simulink library "lib_Convection_MixedIncompFlatPlateBL"  (R2015a)
settings: Solver=ode45  StartTime=0.0  StopTime=10.0  RelTol=1e-3
libraries: lib_Convection_LamIncompFlatPlateBL x1
settings Model: Creator=jlkratz  LastModifiedBy=jlkratz

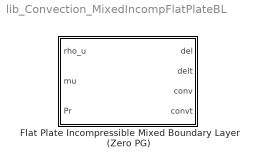
== system lib_Convection_MixedIncompFlatPlateBL ==
  Flat Plate Incompressible Mixed Boundary Layer (Zero PG) : Subsystem  mask(TSAT: Flat Plate Incompressible Mixed Boundary Layer (Zero PG)){x_M=[0.01:0.1:5], BN_M=double(gcb), Retr_M=5000000, xtrip_M=inf}
      mask prompts: x_M "x_M - Local position from the leading edge"; BN_M "BN_M - Block Name"; Retr_M "Retr_M - Transition Reynolds number"; xtrip_M "xtrip_M - Location of a boundary layer trip (inf if none exists)"
      mask help:
      | This block approximates the boundary layer and thermal boundary layer thicknesses of incompressible mixed flow over a flat plate with a pressure gradient of 0. It determines the transition location by the transition Reynolds number or a trip location, whichever is closer to the leading edge. The boundary layer upstream of the transition location is calculated based on the laminar boundary layer solution while downstream the turbulent solution is used. The turbulent solution is shifted such that it intersects the laminar solution at the transition location.
      |
      | For more information see the block help menu.
      mask Help: web(which('Convection_TSAT_MixedIncompFlatPlateBL.html'),'-helpbrowser')
      mask DialogControl Container3 Prompt: Parameters
      mask DialogControl Container5 Prompt: Transition

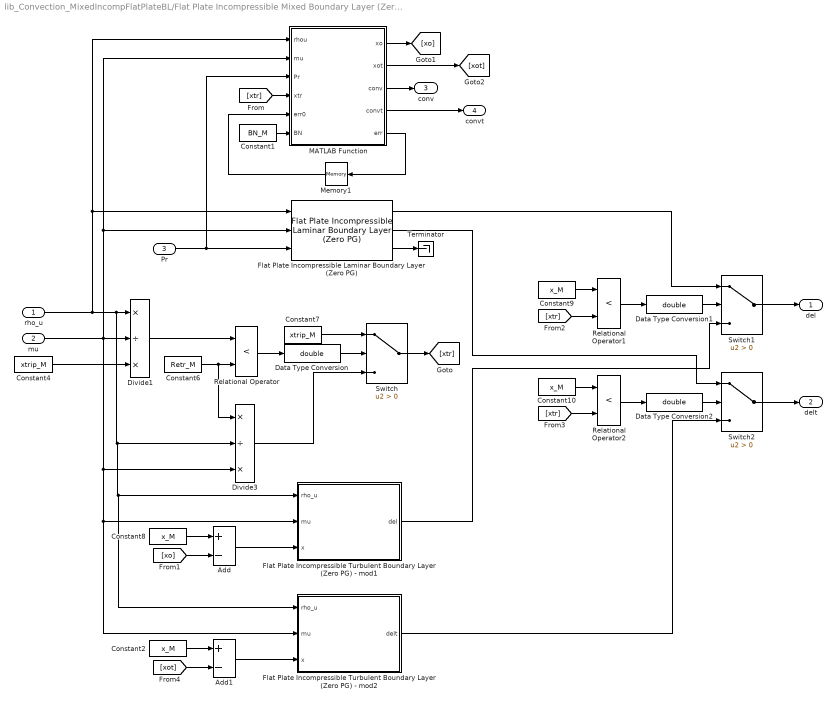
== system lib_Convection_MixedIncompFlatPlateBL/Flat Plate Incompressible Mixed Boundary Layer (Zero PG) ==
  rho_u : Inport
  mu : Inport  Port=2
  Pr : Inport  Port=3
  Add : Sum  Inputs=+-
  Add1 : Sum  Inputs=+-
  Constant1 : Constant  Value=BN_M
  Constant{2,8..10} (4 alike) : Constant  Value=x_M
  Constant4 : Constant  Value=xtrip_M
  Constant6 : Constant  Value=Retr_M
  Constant7 : Constant  Value=xtrip_M
  Data Type Conversion : DataTypeConversion  OutDataTypeStr=double
  Data Type Conversion1 : DataTypeConversion  OutDataTypeStr=double
  Data Type Conversion2 : DataTypeConversion  OutDataTypeStr=double
  Divide1 : Product  Inputs=*/*
  Divide3 : Product  Inputs=*/*
  Flat Plate Incompressible Laminar Boundary Layer (Zero PG) : lib_Convection_LamIncompFlatPlateBL/Flat Plate Incompressible  Laminar Boundary Layer (Zero PG)  Retr_M=Retr_M  x_M=x_M
  Flat Plate Incompressible Turbulent Boundary Layer (Zero PG) - mod1 : Subsystem  mask(TSAT: Flat Plate Incompressible Turbulent Boundary Layer (Zero PG)){x_M=1}
      mask prompts: x_M "x_M - Local position from the leading edge"
      mask help: This block approximates the boundary layer and thermal boundary layer thicknesses of incompressible turbulent flow over a flat plate with a pressure gradient of 0.
      mask Help: web(which('Convection_TSAT_TurbIncompFlatPlateBL.html'),'-helpbrowser')
      mask DialogControl Container3 Prompt: Parameters
  Flat Plate Incompressible Turbulent Boundary Layer (Zero PG) - mod2 : Subsystem  mask(TSAT: Flat Plate Incompressible Turbulent Boundary Layer (Zero PG)){x_M=1}
      mask prompts: x_M "x_M - Local position from the leading edge"
      mask help: This block approximates the boundary layer and thermal boundary layer thicknesses of incompressible turbulent flow over a flat plate with a pressure gradient of 0.
      mask Help: web(which('Convection_TSAT_TurbIncompFlatPlateBL.html'),'-helpbrowser')
      mask DialogControl Container3 Prompt: Parameters
  MATLAB Function : MATLAB Function  TreatAsAtomicUnit=on
  Memory1 : Memory  X0=zeros(1,9)
  Relational Operator : RelationalOperator  Operator=<  OutDataTypeStr=boolean
  Relational Operator1 : RelationalOperator  Operator=<  OutDataTypeStr=boolean
  Relational Operator2 : RelationalOperator  Operator=<  OutDataTypeStr=boolean
  Switch : Switch  Criteria=u2 > Threshold
  Switch1 : Switch  Criteria=u2 > Threshold
  Switch2 : Switch  Criteria=u2 > Threshold
  Terminator : Terminator
  del : Outport
  delt : Outport  Port=2
  conv : Outport  Port=3
  convt : Outport  Port=4
  wires:
  Add1/1 -> Flat Plate Incompressible Turbulent Boundary Layer (Zero PG) - mod2/3(x)
  [xot] -> Add1/2
  Constant2/1 -> Add1/1
  MATLAB Function/4(convt) -> convt/1
  MATLAB Function/2(xot) -> [xot]
  Memory1/1 -> MATLAB Function/5(err0)
  MATLAB Function/3(conv) -> conv/1
  MATLAB Function/1(xo) -> [xo]
  [xtr] -> MATLAB Function/4(xtr)
  Constant1/1 -> MATLAB Function/6(BN)
  MATLAB Function/5(err) -> Memory1/1
  Switch2/1 -> delt/1
  Switch1/1 -> del/1
  Flat Plate Incompressible Turbulent Boundary Layer (Zero PG) - mod2/1(delt) -> Switch2/3
  Flat Plate Incompressible Turbulent Boundary Layer (Zero PG) - mod1/1(del) -> Switch1/3
  Flat Plate Incompressible Laminar Boundary Layer (Zero PG)/2 -> Switch2/1
  [xtr] -> Relational Operator2/2
  Constant10/1 -> Relational Operator2/1
  Relational Operator2/1 -> Data Type Conversion2/1
  Data Type Conversion2/1 -> Switch2/2
  Flat Plate Incompressible Laminar Boundary Layer (Zero PG)/1 -> Switch1/1
  [xtr] -> Relational Operator1/2
  Constant9/1 -> Relational Operator1/1
  Relational Operator1/1 -> Data Type Conversion1/1
  Data Type Conversion1/1 -> Switch1/2
  Add/1 -> Flat Plate Incompressible Turbulent Boundary Layer (Zero PG) - mod1/3(x)
  [xo] -> Add/2
  Constant8/1 -> Add/1
  Flat Plate Incompressible Laminar Boundary Layer (Zero PG)/3 -> Terminator/1
  Pr/1 -> Flat Plate Incompressible Laminar Boundary Layer (Zero PG)/3, MATLAB Function/3(Pr)
  Divide3/1 -> Switch/3
  Switch/1 -> [xtr]
  Constant7/1 -> Switch/1
  Data Type Conversion/1 -> Switch/2
  Relational Operator/1 -> Data Type Conversion/1
  Constant6/1 -> Relational Operator/2, Divide3/1
  Divide1/1 -> Relational Operator/1
  Constant4/1 -> Divide1/3
  mu/1 -> Divide3/3, Flat Plate Incompressible Turbulent Boundary Layer (Zero PG) - mod1/2(mu), Flat Plate Incompressible Turbulent Boundary Layer (Zero PG) - mod2/2(mu), Flat Plate Incompressible Laminar Boundary Layer (Zero PG)/2, MATLAB Function/2(mu), Divide1/2
  rho_u/1 -> Flat Plate Incompressible Laminar Boundary Layer (Zero PG)/1, MATLAB Function/1(rhou), Divide1/1, Divide3/2, Flat Plate Incompressible Turbulent Boundary Layer (Zero PG) - mod1/1(rho_u), Flat Plate Incompressible Turbulent Boundary Layer (Zero PG) - mod2/1(rho_u)

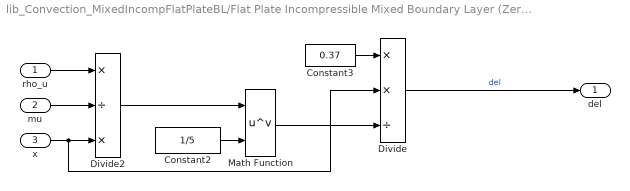
== system lib_Convection_MixedIncompFlatPlateBL/Flat Plate Incompressible Mixed Boundary Layer (Zero PG)/Flat Plate Incompressible Turbulent Boundary Layer (Zero PG) - mod1 ==
  rho_u : Inport
  mu : Inport  Port=2
  x : Inport  Port=3
  Constant2 : Constant  Value=1/5
  Constant3 : Constant  Value=0.37
  Divide : Product  Inputs=**/
  Divide2 : Product  Inputs=*/*
  Math Function : Math  Operator=pow  SaturateOnIntegerOverflow=on
  del : Outport
  wires:
  Divide2/1 -> Math Function/1
  mu/1 -> Divide2/2
  rho_u/1 -> Divide2/1
  x/1 -> Divide2/3, Divide/2
  Constant3/1 -> Divide/1
  Constant2/1 -> Math Function/2
  Math Function/1 -> Divide/3
  Divide/1 -> del/1  "del"

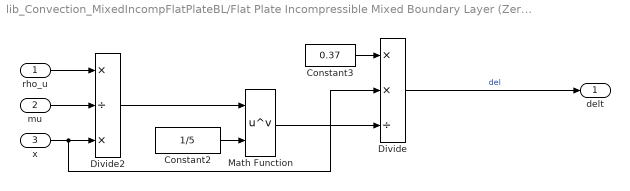
== system lib_Convection_MixedIncompFlatPlateBL/Flat Plate Incompressible Mixed Boundary Layer (Zero PG)/Flat Plate Incompressible Turbulent Boundary Layer (Zero PG) - mod2 ==
  rho_u : Inport
  mu : Inport  Port=2
  x : Inport  Port=3
  Constant2 : Constant  Value=1/5
  Constant3 : Constant  Value=0.37
  Divide : Product  Inputs=**/
  Divide2 : Product  Inputs=*/*
  Math Function : Math  Operator=pow  SaturateOnIntegerOverflow=on
  delt : Outport
  wires:
  Divide/1 -> delt/1  "del"
  Math Function/1 -> Divide/3
  Constant2/1 -> Math Function/2
  Constant3/1 -> Divide/1
  x/1 -> Divide/2, Divide2/3
  rho_u/1 -> Divide2/1
  mu/1 -> Divide2/2
  Divide2/1 -> Math Function/1

== matlab function lib_Convection_MixedIncompFlatPlateBL/Flat Plate Incompressible Mixed Boundary Layer (Zero PG)/MATLAB Function ==
  data: rhou input; xo output; xot output; mu input; Pr input; xtr input; err0 input; BN input; conv output; convt output; err output
function [xo,xot,conv,convt,err] = TransitionXo(rhou,mu,Pr,xtr,err0,BN)
%#codegen

%Warning/Error Check
err = err0;
errNum = 1;
%rhou is a scalar?
if max(size(rhou)) ~= 1 && err0(errNum) ~= 1
    fprintf('warning in %s: rho_u must be a scalar\n',char(BN));
    err(errNum) = 1;
end
errNum = errNum + 1;
%mu is a scalar?
if min(size(mu)) ~= 1 && err0(errNum) ~= 1
    fprintf('warning in %s: mu must be a scalar\n',char(BN));
    err(errNum) = 1;
end
errNum = errNum + 1;
%xtr is a scalar?
if min(size(xtr)) ~= 1 && err0(errNum) ~= 1
    fprintf('warning in %s: xtr must be a scalar\n',char(BN));
    err(errNum) = 1;
end
errNum = errNum + 1;
%rhou is real positive?
if (isreal(rhou) ~= 1 || rhou < 0) && err0(errNum) ~= 1
    fprintf('warning in %s: rho_u must be a real positive number\n',char(BN));
    err(errNum) = 1;
end
errNum = errNum + 1;
%mu is real positive?
if (isreal(mu) ~= 1 || mu < 0) && err0(errNum) ~= 1
    fprintf('warning in %s: mu must be a real positive number\n',char(BN));
    err(errNum) = 1;
end
errNum = errNum + 1;
%xtr is real positive?
if (isreal(xtr) ~= 1 || xtr < 0) && err0(errNum) ~= 1
    fprintf('warning in %s: xtr must be a real positive number\n',char(BN));
    err(errNum) = 1;
end
errNum = errNum + 1;
%rhou has all finite elements?
if (isnan(rhou) > 0 || isinf(rhou) > 0) && err0(errNum) ~= 1
    fprintf('warning in %s: rho_u must have finite value\n',char(BN));
    err(errNum) = 1;
end
errNum = errNum + 1;
%eoD has all finite elements?
if (isnan(mu) > 0 || isinf(mu) > 0) && err0(errNum) ~= 1
    fprintf('warning in %s: mu must have finite value\n',char(BN));
    err(errNum) = 1;
end
%eoD has all finite elements?
if (isnan(xtr) > 0 || isinf(xtr) > 0) && err0(errNum) ~= 1
    fprintf('warning in %s: xtr must have finite value\n',char(BN));
    err(errNum) = 1;
end

%Solve the Colebrook Correlation using the Secant Root Method
Err = 0.000001;
imax = 1000;

%Boundary Layer
Xa = 0.79*xtr;
Xb = 0.83*xtr;
conv = 0;
Xs = 0;
for i = 1:imax %Number iterations is specified by user
    FunXb = 5*xtr*(rhou*xtr/mu)^(-1/2) - 0.37*(xtr-Xb)*(rhou*(xtr-Xb)/mu)^(-1/5); %Value function at Xb is calculated
    FunXa = 5*xtr*(rhou*xtr/mu)^(-1/2) - 0.37*(xtr-Xa)*(rhou*(xtr-Xa)/mu)^(-1/5); %Value function at Xa is calculated
    Xi = Xb - FunXb*(Xa-Xb)/(FunXa-FunXb); %defines new solution by secant method
    %Avoid negative xo
    if Xi <= 0
        Xi = Xa/100;
    end
    if abs((Xi - Xb)/Xb) < Err %if error specification is met Xs is found and loop ends
        Xs = Xi;
        conv = 1;
        break
    end
    Xa = Xb; %if error in solution is not met Xa become Xb
    Xb = Xi; %and Xb become Xi for next iteration
end
if i == imax %if an acceptable solution is not found in imax iteration, and error message is displayed
    conv = 0;
end
xo = Xs;

%Thermal Boundary Layer
Xa = 0.75*xtr;
Xb = 0.79*xtr;
convt = 0;
Xs = 0;
for i = 1:imax %Number iterations is specified by user
    FunXb = 5*xtr*(rhou*xtr/mu)^(-1/2)*Pr^(-0.4) - 0.37*(xtr-Xb)*(rhou*(xtr-Xb)/mu)^(-1/5); %Value function at Xb is calculated
    FunXa = 5*xtr*(rhou*xtr/mu)^(-1/2)*Pr^(-0.4) - 0.37*(xtr-Xa)*(rhou*(xtr-Xa)/mu)^(-1/5); %Value function at Xa is calculated
    Xi = Xb - FunXb*(Xa-Xb)/(FunXa-FunXb); %defines new solution by secant method
    %Avoid negative xo
    if Xi <= 0
        Xi = Xa/100;
    end
    if abs((Xi - Xb)/Xb) < Err %if error specification is met Xs is found and loop ends
        Xs = Xi;
        convt = 1;
        break
    end
    Xa = Xb; %if error in solution is not met Xa become Xb
    Xb = Xi; %and Xb become Xi for next iteration
end
if i == imax %if an acceptable solution is not found in imax iteration, and error message is displayed
    convt = 0;
end
xot = Xs;
